simulink model "Refined_Model_45_Autofactor_GPS"  (R2020b)
settings: Solver=FixedStepAuto  StartTime=0.0  StopTime=2000  FixedStep=dt  RelTol=1e-3
values from neighbouring files (symbols this model uses):
  ALInpSpeed = AxlLoss (1,:)    [ICEBEV_Script_GPS.m]    (also in ICE_Script_GPS.m)
  ALInpTor = AxlLoss(:,1)    [ICEBEV_Script_GPS.m]    (also in ICE_Script_GPS.m)
  ALTableVal = AxlLoss(2:end,2:end)    [ICEBEV_Script_GPS.m]    (also in ICE_Script_GPS.m)
  CF = 0.002408    [ICEBEV_Script_GPS.m]    (also in ICE_Script_GPS.m = VehicleDefine(29,3))
  Cx = VehicleDefine(7,3)    [BEV_Script_GPS.m]    (also in ICEBEV_Script_GPS.m; ICE_Script_GPS.m)
  Dist = [1:length(FMSP1)]    [BEV_Script_GPS.m]    (also in ICEBEV_Script_GPS.m; ICE_Script_GPS.m)
  dt = 0.1    [ICEBEV_Script_GPS.m]    (also in ICE_Script_GPS.m)
  DynRolRad = VehicleDefine(5,3)    [BEV_Script_GPS.m]    (also in ICEBEV_Script_GPS.m; ICE_Script_GPS.m)
  EngineRpm = round(IntpTorCur(:,1))    [ICEBEV_Script_GPS.m]    (also in ICE_Script_GPS.m)
  EngineRpmRaw = TorCurRaw(:,1)    [ICEBEV_Script_GPS.m]    (also in ICE_Script_GPS.m)
  etaClutch = VehicleDefine(23,3)    [ICEBEV_Script_GPS.m]    (also in ICE_Script_GPS.m)
  FCMap = xlsread('C:\Users\Kshitij\Desktop\Thesis docs\Code\Total Simulink  Model files\Vehicle 6 - Class 5 tractorEtrailer\FC_Map.xlsx')    [ICEBEV_Script_GPS.m]    (also in ICE_Script_GPS.m = xlsread('C:\Users\Kshitij\Desktop\Thesis docs\Code\Total Sim)
  FCTableVal = FCMap(2:end,2:end)    [ICEBEV_Script_GPS.m]    (also in ICE_Script_GPS.m)
  FDR = VehicleDefine(20,3)    [BEV_Script_GPS.m]    (also in ICEBEV_Script_GPS.m = VehicleDefine(22,3); ICE_Script_GPS.m = VehicleDefine(22,3))
  FMSP1 = FMSP    [BEV_Script_GPS.m]    (also in ICEBEV_Script_GPS.m; ICE_Script_GPS.m)
  Fr = VehicleDefine(13,3)    [BEV_Script_GPS.m]    (also in ICEBEV_Script_GPS.m; ICE_Script_GPS.m)
  g = VehicleDefine(14,3)    [BEV_Script_GPS.m]    (also in ICEBEV_Script_GPS.m; ICE_Script_GPS.m)
  GearNo = unique(GLoss(:,1))    [GearLossMap.m]
  GNo = GBXDefine(:,1)    [ICEBEV_Script_GPS.m]    (also in ICE_Script_GPS.m)
  GRa = GBXDefine(:,2)    [ICEBEV_Script_GPS.m]    (also in ICE_Script_GPS.m)
  IntpSlope = round(IntpSlope,1)    [BEV_Script_GPS.m]    (also in ICEBEV_Script_GPS.m; ICE_Script_GPS.m)
  Je = VehicleDefine(25,3)    [ICEBEV_Script_GPS.m]    (also in ICE_Script_GPS.m)
  Jk = VehicleDefine(15,3)    [BEV_Script_GPS.m]    (also in ICEBEV_Script_GPS.m = Etr(1,3); ICE_Script_GPS.m)
  Jm = VehicleDefine(16,3)    [ICEBEV_Script_GPS.m]    (also in ICE_Script_GPS.m)
  MaxAcc = 1    [BEV_Script_GPS.m]    (also in ICEBEV_Script_GPS.m; ICE_Script_GPS.m)
  MaxDec = 1    [BEV_Script_GPS.m]    (also in ICEBEV_Script_GPS.m; ICE_Script_GPS.m)
  MaxTorValThrot = max(ThrotTableVal,[],2)    [ICEBEV_Script_GPS.m]    (also in ICE_Script_GPS.m)
  Me = VehicleDefine(10,3)    [BEV_Script_GPS.m]    (also in ICEBEV_Script_GPS.m; ICE_Script_GPS.m)
  MotoringTor = IntpTorCur(:,3)    [ICEBEV_Script_GPS.m]    (also in ICE_Script_GPS.m)
  Mt = VehicleDefine(12,3)    [BEV_Script_GPS.m]    (also in ICEBEV_Script_GPS.m; ICE_Script_GPS.m)
  Mtot = Mv+Me+Mt    [BEV_Script_GPS.m]    (also in ICEBEV_Script_GPS.m; ICE_Script_GPS.m)
  Mv = VehicleDefine(9,3)    [BEV_Script_GPS.m]    (also in ICEBEV_Script_GPS.m; ICE_Script_GPS.m)
  NoSteps = (round(Dist(end))+3)    [BEV_Script_GPS.m]    (also in ICEBEV_Script_GPS.m; ICE_Script_GPS.m; VectoSPpm.m = max(D))
  NoWhl = VehicleDefine(2,3)    [ICEBEV_Script_GPS.m]    (also in ICE_Script_GPS.m)
  NoWhlDri = VehicleDefine(4,3)    [ICEBEV_Script_GPS.m]    (also in ICE_Script_GPS.m)
  PTOF = 0.003255    [ICEBEV_Script_GPS.m]    (also in ICE_Script_GPS.m = VehicleDefine(28,3))
  rho = VehicleDefine(6,3)    [BEV_Script_GPS.m]    (also in ICEBEV_Script_GPS.m; ICE_Script_GPS.m)
  RpmBrkPnt = ThrottleMap(1,:)    [ICEBEV_Script_GPS.m]    (also in ICE_Script_GPS.m)
  s = divisors(length(MaxSpeedProfile))    [BEV_Script_GPS.m]    (also in ICEBEV_Script_GPS.m; ICE_Script_GPS.m; interparc.m = totalsplinelength*t)
  SegSPLatinmps = (sqrt(aMaxLat*g*CurRadinm))    [BEV_Script_GPS.m]    (also in ICEBEV_Script_GPS.m; ICE_Script_GPS.m)
  Stoptimes = readmatrix('C:\Users\Kshitij\Desktop\Thesis docs\Code\Total Simulink  Model files\GPS Routes and OC\Turin - Lyon - OC_description.xlsx','Sheet','Stop')    [BEV_Script_GPS.m]    (also in ICEBEV_Script_GPS.m; ICE_Script_GPS.m)
  Sx = VehicleDefine(8,3)    [BEV_Script_GPS.m]    (also in ICEBEV_Script_GPS.m; ICE_Script_GPS.m)
  ThrotPos = ThrotPos'    [ICEBEV_Script_GPS.m]    (also in ICE_Script_GPS.m)
  ThrotTableVal = ThrottleMap(2:end,2:end)    [ICEBEV_Script_GPS.m]    (also in ICE_Script_GPS.m)
undefined symbols (not defined in the file or in its folder): CovDist, G1Inprpm, GInprpm, GInpTor, GTorLoss, MaxSpinG, MaxWhlTorinG, SegNo
libraries: simulink x5, autolibshared x1
(part 2 of 2)

== system Refined_Model_45_Autofactor_GPS/ICE Vehicle model/Engine Model/Engine Idling/If Action Subsystem1 ==
  In1 : Inport
  Action Port : ActionPort  ActionPortLabel=else
  Out1 : Outport
  wires:
  In1/1 -> Out1/1

== system Refined_Model_45_Autofactor_GPS/Driver Model/Gear and Clutch Definition/Clutch position definition/Triggered Single Pulse/+ve edge detect ==
  note: Edge
  signal : Inport
  Delay Input1 : UnitDelay  Description=Store in Global RAM  DisableCoverage=on  SampleTime=-1  HasFrameUpgradeWarning=on
  FixPt Relational Operator : RelationalOperator  Operator=>  OutDataTypeStr=fixdt(0, 8)  ZeroCross=off  RndMeth=Nearest
  Positive : simulink/Logic and Bit Operations/Compare To Zero  relop=>  OutDataTypeStr=uint8  ZeroCross=off
  out : Outport
  wires:
  Delay Input1/1 -> FixPt Relational Operator/2  "U(k-1)"
  Positive/1 -> Delay Input1/1, FixPt Relational Operator/1  "U(k)"
  FixPt Relational Operator/1 -> out/1
  signal/1 -> Positive/1

== stateflow chart Refined_Model_45_Autofactor_GPS/Driver Model/Acc//Dec Control/Driving State ==
  state PTO_limiting
    Factor = PTOFactor;
    idle = 0;
    Bor = 0;
    Aor = 1;
    error = x;
  state Stopping
    Factor = 0;
    idle = 0;
    Bor = 1;
    Aor = 0;
    error = x;
  state Driving
    idle = 0;
    Bor = 0;
    Aor = 1;
    error = x;
    Factor = CoastingFactor;
  state Idling
    Factor = 0;
    idle = 1;
    Bor = 1;
    Aor = 0;
    error = x;
  state Calibration_pve
    Factor = 0;
    idle = 1;
    Bor = 1;
    Aor = 0;
    x = Dist2NStop;
  state Calibration_nve
    Factor = 0;
    idle = 1;
    Bor = 1;
    Aor = 0;
    x = Dist2PStop;
  PTO_limiting -> Driving : [v >= vtarg && a <= 0.01]
  Driving -> PTO_limiting [order 2] : [v <= 1 && a > 0]
  Stopping -> Calibration_nve [order 2] : [v == 0 && d > 0 && Dist2PStop <= 25 && Dist2Dec <= 0]{Bor = 1;}
  (default) -> Driving : {x = 0; Factor = 0;}
  Driving -> Stopping [order 1] : [Dist2NStop <= Dist2Dec && UpSp <= 1]
  Idling -> Driving : after(Stoptime/3.7,sec) [a == 0]{Aor == 1}
  Stopping -> Calibration_pve [order 1] : [v == 0 && d > 0 && Dist2NStop <= 25 && Dist2Dec == 0]{Bor = 1;}
  Calibration_pve -> Idling : [v == 0]{idle = 1;Bor = 1;x = x + Dist2NStop}
  Calibration_nve -> Idling : [v == 0 ]{idle = 1;Bor = 1;x = x - Dist2PStop}
  data: x output double; v input; a input; d input; idle output =0; Bor output; Stoptime input; Dist2NStop input; Dist2Dec input; UpSp input; Dist2PStop input; Aor output; error local; Factor output; vtarg input; PTOFactor input; CoastingFactor input
